simulink model "IntegratedSteamNetworkSimulation"  (R2022b)
settings: Solver=ode4  StartTime=0  StopTime=1000  FixedStep=0.5  MaxStep=1  MinStep=1e-3  EnableMultiTasking=on
values from neighbouring files (symbols this model uses):
  Attemp1_PB = 334.14047    [BoilerParam.m]
  Attemp1_RB = 332.70172955    [BoilerParam.m]
  Attemp2_PB = 426.4464    [BoilerParam.m]
  Attemp2_RB = 423.6721137    [BoilerParam.m]
  Attempflow_init = 0    [BoilerParam.m]
  Attempflow_SS = 11355    [BoilerParam.m]
  Attempflow_SSRB = 2.3*11355    (= 26116.5)    [BoilerParam.m]
  FG_flow_RB = 2.3*FGFlow_SS    (= 420210)    [BoilerParam.m]
  FGFlow_SS = 182700    [BoilerParam.m]
  hf = u(3)    [Boiler3.m]    (also in Boiler4.m; BoilerParam.m = 900000)
  phin = 6.21000008802327    (= 6.21000008802)    [BoilerParam.m]
  qfsteadystate = 73.2301    [BoilerParam.m]
  qfsteadystate2 = 31.5677    [BoilerParam.m]
  Qsteadystate = 1.374070083420811e+008    (= 137407008.342)    [BoilerParam.m]
  Qsteadystate2 = 5.9194e+007    (= 59194000)    [BoilerParam.m]
  TFG_out1_initPB = 432.2968    [BoilerParam.m]
  TFG_out1_initRB = 434.8845734    [BoilerParam.m]
  TFG_out2_initPB = 483.8618    [BoilerParam.m]
  TFG_out2_initRB = 486.31627357    [BoilerParam.m]
  TFG_out3_initPB = 543.7293    [BoilerParam.m]
  TFG_out3_initRB = 545.8638828    [BoilerParam.m]
  TFG_out4_initPB = 611.0105    [BoilerParam.m]
  TFG_out4_initRB = 612.6928895    [BoilerParam.m]
  TFG_out5_initPB = 684.8106    [BoilerParam.m]
  TFG_out5_initRB = 685.9654778    [BoilerParam.m]
  TFG_out6_initPB = 764.5389    [BoilerParam.m]
  TFG_out6_initRB = 765.12376925    [BoilerParam.m]
  Ts_out1_init_PB = 303.33953    [BoilerParam.m]
  Ts_out1_init_RB = 302.2065815    [BoilerParam.m]
  Ts_out2_init_PB = 334.14047    [BoilerParam.m]
  Ts_out2_init_RB = 332.70172955    [BoilerParam.m]
  Ts_out3_init_PB = 375.4672    [BoilerParam.m]
  Ts_out3_init_RB = 373.4655693    [BoilerParam.m]
  Ts_out4_init_PB = 426.4464    [BoilerParam.m]
  Ts_out4_init_RB = 423.6721137    [BoilerParam.m]
  Ts_out5_init_PB = 485.4202    [BoilerParam.m]
  Ts_out5_init_RB = 481.745302    [BoilerParam.m]
  Ts_out6_init_PB = 550.8115    [BoilerParam.m]
  Ts_out6_init_RB = 546.1691598    [BoilerParam.m]
  X0 = [106.953303000225 ... (first row only)    [BoilerParam.m]
  X02 = [39.2837325596915 ... (first row only)    [BoilerParam.m]
undefined symbols (not defined in the file or in its folder): Param, Param2, Param3, Param4, Param5, Param6
libraries: slpidlib x1
(part 1 of 2)
settings Model: Creator=aitai  LastModifiedBy=acer
settings DataIOCC: LimitDataPoints=on  SaveFinalState=on  SaveFormat=StructureWithTime  SignalLoggingSaveFormat=ModelDataLogs  ReturnWorkspaceOutputs=off  Refine=5
settings OptimizationCC: BlockReduction=off  BooleanDataType=off  BufferReuse=off  InitFltsAndDblsToZero=on  LifeSpan=inf
settings DebuggingCC: AlgebraicLoopMsg=none  SaveWithParameterizedLinksMsg=none  UnderspecifiedInitializationDetection=Classic  MergeDetectMultiDrivingBlocksExec=none  SignalResolutionControl=TryResolveAllWithWarning  MultiTaskDSMMsg=warning  MultiTaskCondExecSysMsg=none  SFUnexpectedBacktrackingDiag=warning  SFNoUnconditionalDefaultTransitionDiag=warning  SFExecutionAtInitializationDiag=none  SFMachineParentedDataDiag=warning  ArithmeticOperatorsInVariantConditions=warning
settings HardwareCC: ProdBitPerPointer=32  ProdBitPerSizeT=32  ProdBitPerPtrDiffT=32  ProdLargestAtomicFloat=None  ProdIntDivRoundTo=Undefined  ProdEndianess=Unspecified  ProdWordSize=32  ProdHWDeviceType=32-bit Generic  TargetUnknown=on
settings ModelReferenceCC: EnableRefExpFcnMdlSchedulingChecks=on  PropagateSignalLabelsOutOfModel=off
settings RTWCC: DLArmComputeVersion=19.05
settings CodeAppCC: StateflowObjectComments=on
settings GRTTargetCC: TargetFcnLib=ansi_tfl_tmw.mat  TargetLangStandard=C89/C90 (ANSI)  ModelReferenceCompliant=off  CombineOutputUpdateFcns=off  MatFileLogging=off  GRTInterface=on
settings ConfigComp: CovMetricSettings=dw  CovSaveCumulativeToWorkspaceVar=on  CovSaveSingleToWorkspaceVar=on

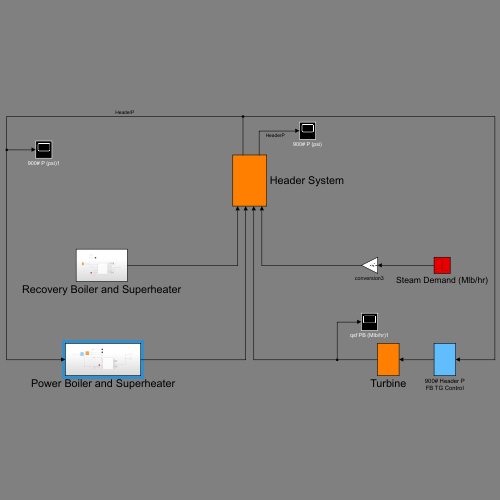
[thumbnail: Simulink's stored preview of the top-level diagram]
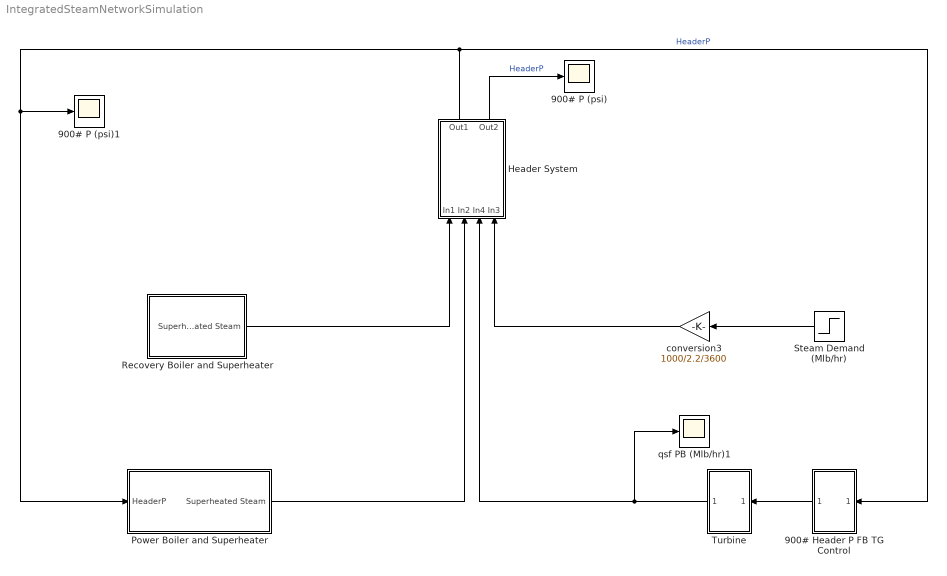
== system IntegratedSteamNetworkSimulation ==
  900# Header P FB TG Control : Subsystem
      mask Display: disp('')
  900# P (psi) : Scope
  900# P (psi)1 : Scope
  Header System : Subsystem
      mask Display: disp('')
  Power Boiler and Superheater : Subsystem
  Recovery Boiler and Superheater : Subsystem
  Steam Demand (Mlb/hr) : Step  Time=50  Before=240  After=210  SampleTime=0  VectorParams1D=off
  Turbine : Subsystem
      mask Display: disp('')
  conversion3 : Gain  Gain=1000/2.2/3600  SaturateOnIntegerOverflow=on  OutDataTypeStr=Inherit: Same as input  ParamDataTypeStr=Inherit: Same as input
  qsf PB (Mlb/hr)1 : Scope
  wires:
  Header System/1(Out1) -> 900# P (psi)1/1, Power Boiler and Superheater/1(HeaderP), 900# Header P FB TG Control/1(In1)  "HeaderP"
  Turbine/1(Out1) -> Header System/3(In4), qsf PB (Mlb/hr)1/1
  Steam Demand (Mlb/hr)/1 -> conversion3/1
  Header System/2(Out2) -> 900# P (psi)/1  "HeaderP"
  conversion3/1 -> Header System/4(In3)
  900# Header P FB TG Control/1(Out1) -> Turbine/1(In1)
  Power Boiler and Superheater/1(Superheated Steam) -> Header System/2(In2)
  Recovery Boiler and Superheater/1(Superheated Steam) -> Header System/1(In1)

== system IntegratedSteamNetworkSimulation/900# Header P FB TG Control ==
  In1 : Inport
  1/Ti1 : Gain  Gain=0.01  SaturateOnIntegerOverflow=on  OutDataTypeStr=Inherit: Same as input  ParamDataTypeStr=Inherit: Same as input
  900#  P Setpoint (psi) : Constant  Value=900
  Integrator1 : Integrator
  Kc1 : Gain  Gain=45  SaturateOnIntegerOverflow=on  OutDataTypeStr=Inherit: Same as input  ParamDataTypeStr=Inherit: Same as input
  P action1 : Gain  SaturateOnIntegerOverflow=on  OutDataTypeStr=Inherit: Same as input  ParamDataTypeStr=Inherit: Same as input
  Real Output from CO : Gain  Gain=0.01  SaturateOnIntegerOverflow=on  OutDataTypeStr=Inherit: Same as input  ParamDataTypeStr=Inherit: Same as input
  Sum2 : Sum  Inputs=|++  InputSameDT=on  SaturateOnIntegerOverflow=on  OutDataTypeStr=Inherit: Same as first input
  Sum3 : Sum  Inputs=|+-  InputSameDT=on  SaturateOnIntegerOverflow=on  OutDataTypeStr=Inherit: Same as first input
  Unit Delay : UnitDelay  SampleTime=-1  HasFrameUpgradeWarning=on
  conversion : Gain  Gain=6.21e6/900  SaturateOnIntegerOverflow=on  OutDataTypeStr=Inherit: Same as input  ParamDataTypeStr=Inherit: Same as input
  error as % of SP : Gain  Gain=100/6.21e6  SaturateOnIntegerOverflow=on  OutDataTypeStr=Inherit: Same as input  ParamDataTypeStr=Inherit: Same as input
  Out1 : Outport
  wires:
  1/Ti1/1 -> Integrator1/1
  Sum2/1 -> Kc1/1
  P action1/1 -> Sum2/1
  Integrator1/1 -> Sum2/2
  error as % of SP/1 -> 1/Ti1/1, P action1/1
  Kc1/1 -> Real Output from CO/1
  In1/1 -> Sum3/2
  900#  P Setpoint (psi)/1 -> conversion/1
  Sum3/1 -> error as % of SP/1
  Real Output from CO/1 -> Unit Delay/1
  conversion/1 -> Sum3/1
  Unit Delay/1 -> Out1/1

== system IntegratedSteamNetworkSimulation/Header System ==
  In1 : Inport
  In2 : Inport  Port=2
  In4 : Inport  Port=3
  In3 : Inport  Port=4
  " " : Gain  Gain=1e6  SaturateOnIntegerOverflow=on  OutDataTypeStr=Inherit: Same as input  ParamDataTypeStr=Inherit: Same as input
  Hdr : S-Function  FunctionName=hdr  Parameters=Param,phin  SFunctionDeploymentMode=off  EnableBusSupport=off
  Mux : Mux
  conversion : Gain  Gain=1/6.9e3  SaturateOnIntegerOverflow=on  OutDataTypeStr=Inherit: Same as input  ParamDataTypeStr=Inherit: Same as input
  Out1 : Outport
  Out2 : Outport  Port=2
  wires:
  In1/1 -> Mux/1
  In2/1 -> Mux/2
  In3/1 -> Mux/3
  In4/1 -> Mux/4
  Hdr/1 -> " "/1
  Mux/1 -> Hdr/1  "kg/s"
  " "/1 -> Out1/1, conversion/1  "Pa"
  conversion/1 -> Out2/1  "Psil"

== system IntegratedSteamNetworkSimulation/Power Boiler and Superheater ==
  note: s
  HeaderP : Inport
  900# Header P FB PB Control : Subsystem
      mask Display: disp('')
  FG Flow : Step  Before=FGFlow_SS  After=FGFlow_SS  SampleTime=0
  FG Temp : Scope  NumInputPorts=6
  Gain : Gain  Gain=FGFlow_SS
  PB Superheater : Subsystem
  Power Boiler : Subsystem
      mask Display: disp('')
  SH Steam Flow : Scope
  SH Steam Temp : Scope  NumInputPorts=8
  Scope6 : Scope
  Sum : Sum  Inputs=|++
  U1 : Step  Time=50000  Before=1.6  After=1.5  SampleTime=0
  conversion2 : Gain  Gain=2.2*3600/1000  SaturateOnIntegerOverflow=on  OutDataTypeStr=Inherit: Same as input  ParamDataTypeStr=Inherit: Same as input
  conversion4 : Gain  Gain=3600  SaturateOnIntegerOverflow=on  OutDataTypeStr=Inherit: Same as input  ParamDataTypeStr=Inherit: Same as input
  qsf PB (Mlb/hr) : Scope
  qsf PB (kg/s) : Scope
  Superheated Steam : Outport
  wires:
  conversion4/1 -> PB Superheater/2(Steamflowboiler)  "kg/hr"
  U1/1 -> PB Superheater/3(U-Value)
  PB Superheater/8(Ts_Out6) -> SH Steam Temp/8
  PB Superheater/9(SteamflowOut SH) -> Superheated Steam/1, SH Steam Flow/1  "Superheated Steam"
  HeaderP/1 -> 900# Header P FB PB Control/1(In1)
  PB Superheater/7(Ts_Out5) -> SH Steam Temp/7
  Power Boiler/1(qsf) -> conversion4/1, qsf PB (kg/s)/1, conversion2/1  "Saturated Steam"
  PB Superheater/6(Ts_OutAttemp2) -> SH Steam Temp/6
  PB Superheater/4(Ts_Out3) -> SH Steam Temp/4
  PB Superheater/13(TFG_Out4) -> FG Temp/4
  PB Superheater/1(Ts_out1) -> SH Steam Temp/1
  PB Superheater/11(TFG_Out2) -> FG Temp/2
  Power Boiler/2(PB_p) -> PB Superheater/1(Boiler Pressure)  "PB_P (Psi)"
  PB Superheater/2(Ts_Out2) -> SH Steam Temp/2
  900# Header P FB PB Control/1(Out1) -> Power Boiler/1(Delta Q)
  conversion2/1 -> qsf PB (Mlb/hr)/1
  PB Superheater/14(TFG_Out5) -> FG Temp/5
  PB Superheater/5(Ts_Out4) -> SH Steam Temp/5
  PB Superheater/10(TFG_Out1) -> FG Temp/1
  FG Flow/1 -> Sum/2
  PB Superheater/3(Ts_OutAttemp1) -> SH Steam Temp/3
  PB Superheater/12(TFG_Out3) -> FG Temp/3
  PB Superheater/15(TFG_Out6) -> FG Temp/6
  900# Header P FB PB Control/2(Output) -> Gain/1
  Sum/1 -> Scope6/1, PB Superheater/4(FG_flow)
  Gain/1 -> Sum/1

== system IntegratedSteamNetworkSimulation/Recovery Boiler and Superheater ==
  FG Flow1 : Step  Before=FG_flow_RB  After=FG_flow_RB  SampleTime=0
  FG Temp : Scope  NumInputPorts=6
  RB Superheater : Subsystem
  Recovery Boiler : Subsystem
      mask Display: disp('')
  SH Steam Temp : Scope  NumInputPorts=8
  Scope2 : Scope
  Scope4 : Scope
  U2 : Step  Time=50000  Before=1.6  After=1.5  SampleTime=0
  conversion1 : Gain  Gain=2.2*3600/1000  SaturateOnIntegerOverflow=on  OutDataTypeStr=Inherit: Same as input  ParamDataTypeStr=Inherit: Same as input
  conversion5 : Gain  Gain=3600  SaturateOnIntegerOverflow=on  OutDataTypeStr=Inherit: Same as input  ParamDataTypeStr=Inherit: Same as input
  qsf RB (Mlb/hr) : Scope
  Superheated Steam : Outport
  wires:
  RB Superheater/14(TFG_Out5) -> FG Temp/5
  Recovery Boiler/1(qsf) -> conversion5/1, Scope2/1, conversion1/1  "Saturated Steam"
  conversion1/1 -> qsf RB (Mlb/hr)/1
  RB Superheater/4(Ts_Out3) -> SH Steam Temp/4
  RB Superheater/15(TFG_Out6) -> FG Temp/6
  RB Superheater/5(Ts_Out4) -> SH Steam Temp/5
  RB Superheater/6(Ts_OutAttemp2) -> SH Steam Temp/6
  RB Superheater/2(Ts_Out2) -> SH Steam Temp/2
  RB Superheater/3(Ts_OutAttemp1) -> SH Steam Temp/3
  RB Superheater/11(TFG_Out2) -> FG Temp/2
  RB Superheater/8(Ts_Out6) -> SH Steam Temp/8
  RB Superheater/7(Ts_Out5) -> SH Steam Temp/7
  RB Superheater/9(SteamflowOut SH) -> Superheated Steam/1, Scope4/1
  conversion5/1 -> RB Superheater/2(Steamflowboiler)  "kg/hr"
  RB Superheater/1(Ts_out1) -> SH Steam Temp/1
  FG Flow1/1 -> RB Superheater/4(FG_flow)
  RB Superheater/13(TFG_Out4) -> FG Temp/4
  RB Superheater/10(TFG_Out1) -> FG Temp/1
  RB Superheater/12(TFG_Out3) -> FG Temp/3
  Recovery Boiler/2(RB_P) -> RB Superheater/1(Boiler Pressure)  "RB_P"
  U2/1 -> RB Superheater/3(U-Value)

== system IntegratedSteamNetworkSimulation/Turbine ==
  In1 : Inport
  Sum4 : Sum  Inputs=|-+  InputSameDT=on  SaturateOnIntegerOverflow=on  OutDataTypeStr=Inherit: Same as first input
  TG Dynamics : TransferFcn  Denominator=[5 1]
  TG SS Demand (Mlb/hr) : Constant  Value=590
  conversion : Gain  Gain=1000/2.2/3600  SaturateOnIntegerOverflow=on  OutDataTypeStr=Inherit: Same as input  ParamDataTypeStr=Inherit: Same as input
  Out1 : Outport
  wires:
  TG SS Demand (Mlb/hr)/1 -> conversion/1
  TG Dynamics/1 -> Sum4/1
  Sum4/1 -> Out1/1
  In1/1 -> TG Dynamics/1
  conversion/1 -> Sum4/2

== system IntegratedSteamNetworkSimulation/Power Boiler and Superheater/900# Header P FB PB Control ==
  In1 : Inport
  1/Ti1 : Gain  Gain=0.001  SaturateOnIntegerOverflow=on  OutDataTypeStr=Inherit: Same as input  ParamDataTypeStr=Inherit: Same as input
  900#  P Setpoint (psi) : Constant  Value=900
  Constant : Constant  Value=Qsteadystate2
  Divide : Product  Inputs=*/
  Integrator1 : Integrator
  Kc1 : Gain  Gain=15  SaturateOnIntegerOverflow=on  OutDataTypeStr=Inherit: Same as input  ParamDataTypeStr=Inherit: Same as input
  P action1 : Gain  SaturateOnIntegerOverflow=on  OutDataTypeStr=Inherit: Same as input  ParamDataTypeStr=Inherit: Same as input
  Real Output from CO : Gain  Gain=Qsteadystate2/100  SaturateOnIntegerOverflow=on  OutDataTypeStr=Inherit: Same as input  ParamDataTypeStr=Inherit: Same as input
  Scope : Scope  NumInputPorts=2
  Scope1 : Scope
  Sum2 : Sum  Inputs=|++  InputSameDT=on  SaturateOnIntegerOverflow=on  OutDataTypeStr=Inherit: Same as first input
  Sum3 : Sum  Inputs=|+-  InputSameDT=on  SaturateOnIntegerOverflow=on  OutDataTypeStr=Inherit: Same as first input
  conversion : Gain  Gain=6.21e6/900  SaturateOnIntegerOverflow=on  OutDataTypeStr=Inherit: Same as input  ParamDataTypeStr=Inherit: Same as input
  error as % of SP : Gain  Gain=100/6.21e6  SaturateOnIntegerOverflow=on  OutDataTypeStr=Inherit: Same as input  ParamDataTypeStr=Inherit: Same as input
  Out1 : Outport
  Output : Outport  Port=2
  wires:
  1/Ti1/1 -> Integrator1/1
  Sum2/1 -> Kc1/1
  P action1/1 -> Sum2/1
  Integrator1/1 -> Sum2/2
  error as % of SP/1 -> 1/Ti1/1, P action1/1
  Kc1/1 -> Scope/1, Real Output from CO/1
  In1/1 -> Sum3/2
  900#  P Setpoint (psi)/1 -> conversion/1
  Sum3/1 -> error as % of SP/1
  Real Output from CO/1 -> Divide/1, Out1/1, Scope/2
  conversion/1 -> Sum3/1
  Constant/1 -> Divide/2
  Divide/1 -> Scope1/1, Output/1

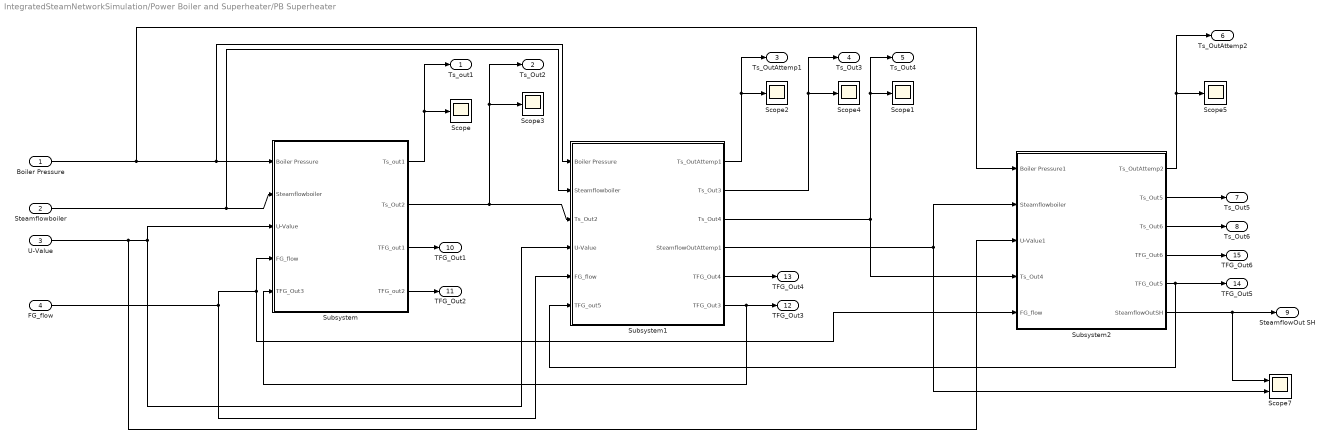
== system IntegratedSteamNetworkSimulation/Power Boiler and Superheater/PB Superheater ==
  Boiler Pressure : Inport
  Steamflowboiler : Inport  Port=2
  U-Value : Inport  Port=3
  FG_flow : Inport  Port=4
  Scope{,1..5} (6 alike) : Scope
  Scope7 : Scope  NumInputPorts=2
  Subsystem : Subsystem
  Subsystem1 : Subsystem
  Subsystem2 : Subsystem
  Ts_out1 : Outport
  Ts_Out2 : Outport  Port=2
  Ts_OutAttemp1 : Outport  Port=3
  Ts_Out3 : Outport  Port=4
  Ts_Out4 : Outport  Port=5
  Ts_OutAttemp2 : Outport  Port=6
  Ts_Out5 : Outport  Port=7
  Ts_Out6 : Outport  Port=8
  SteamflowOut SH : Outport  Port=9
  TFG_Out1 : Outport  Port=10
  TFG_Out2 : Outport  Port=11
  TFG_Out3 : Outport  Port=12
  TFG_Out4 : Outport  Port=13
  TFG_Out5 : Outport  Port=14
  TFG_Out6 : Outport  Port=15
  wires:
  Subsystem/1(Ts_out1) -> Ts_out1/1, Scope/1
  Steamflowboiler/1 -> Subsystem1/2(Steamflowboiler), Subsystem/2(Steamflowboiler)
  Boiler Pressure/1 -> Subsystem2/1(Boiler Pressure1), Subsystem/1(Boiler Pressure), Subsystem1/1(Boiler Pressure)
  Subsystem/2(Ts_Out2) -> Subsystem1/3(Ts_Out2), Ts_Out2/1, Scope3/1
  Subsystem1/1(Ts_OutAttemp1) -> Ts_OutAttemp1/1, Scope2/1
  Subsystem1/2(Ts_Out3) -> Ts_Out3/1, Scope4/1
  Subsystem1/3(Ts_Out4) -> Scope1/1, Ts_Out4/1, Subsystem2/4(Ts_Out4)
  U-Value/1 -> Subsystem2/3(U-Value1), Subsystem1/4(U-Value), Subsystem/3(U-Value)
  Subsystem2/1(Ts_OutAttemp2) -> Scope5/1, Ts_OutAttemp2/1
  Subsystem2/2(Ts_Out5) -> Ts_Out5/1
  Subsystem2/3(Ts_Out6) -> Ts_Out6/1
  Subsystem2/6(SteamflowOutSH) -> Scope7/1, SteamflowOut SH/1
  Subsystem1/4(SteamflowOutAttemp1) -> Subsystem2/2(Steamflowboiler), Scope7/2
  FG_flow/1 -> Subsystem2/5(FG_flow), Subsystem/4(FG_flow), Subsystem1/5(FG_flow)
  Subsystem1/6(TFG_Out3) -> Subsystem/5(TFG_Out3), TFG_Out3/1
  Subsystem2/5(TFG_Out5) -> Subsystem1/6(TFG_out5), TFG_Out5/1
  Subsystem/3(TFG_out1) -> TFG_Out1/1
  Subsystem/4(TFG_out2) -> TFG_Out2/1
  Subsystem1/5(TFG_Out4) -> TFG_Out4/1
  Subsystem2/4(TFG_Out6) -> TFG_Out6/1

== system IntegratedSteamNetworkSimulation/Power Boiler and Superheater/Power Boiler ==
  Delta Q : Inport
  3 Element Level Control System : Subsystem
  PB feed water (Mlb/hr) : Scope
  PB level (in) : Scope
  PB pressure (psi) : Scope
  Power Boiler : Subsystem
  qsf : Outport
  PB_p : Outport  Port=2
  wires:
  Power Boiler/2(qsf) -> qsf/1, 3 Element Level Control System/2(In2)
  Power Boiler/1(l) -> PB level (in)/1, 3 Element Level Control System/1(In1)
  Delta Q/1 -> Power Boiler/2(Delta Q)
  Power Boiler/3(PB p) -> PB_p/1, PB pressure (psi)/1
  Power Boiler/4(qf) -> PB feed water (Mlb/hr)/1
  3 Element Level Control System/1(Delta qf) -> Power Boiler/1(Delta qf)

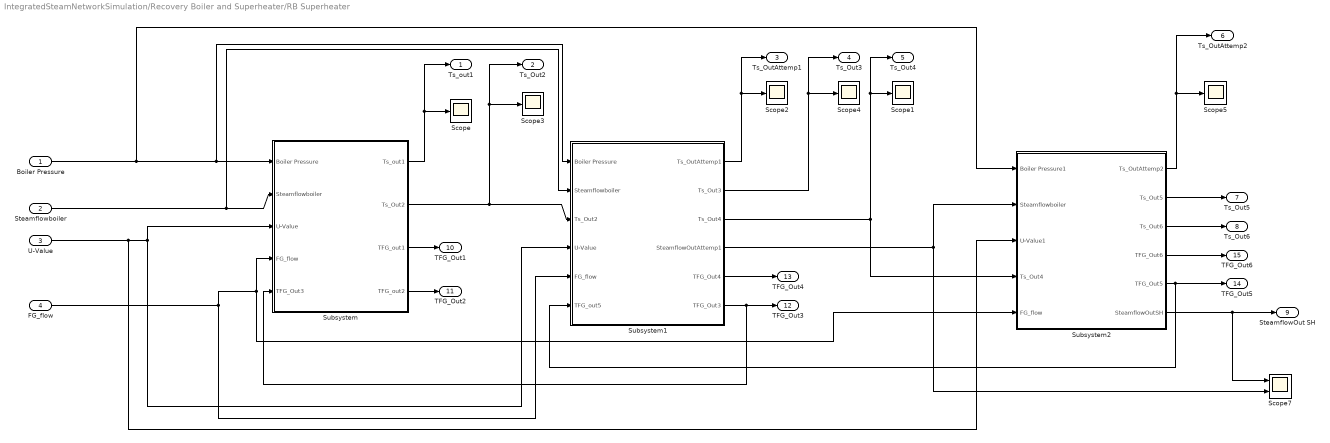
== system IntegratedSteamNetworkSimulation/Recovery Boiler and Superheater/RB Superheater ==
  Boiler Pressure : Inport
  Steamflowboiler : Inport  Port=2
  U-Value : Inport  Port=3
  FG_flow : Inport  Port=4
  Scope{,1..5} (6 alike) : Scope
  Scope7 : Scope  NumInputPorts=2
  Subsystem : Subsystem
  Subsystem1 : Subsystem
  Subsystem2 : Subsystem
  Ts_out1 : Outport
  Ts_Out2 : Outport  Port=2
  Ts_OutAttemp1 : Outport  Port=3
  Ts_Out3 : Outport  Port=4
  Ts_Out4 : Outport  Port=5
  Ts_OutAttemp2 : Outport  Port=6
  Ts_Out5 : Outport  Port=7
  Ts_Out6 : Outport  Port=8
  SteamflowOut SH : Outport  Port=9
  TFG_Out1 : Outport  Port=10
  TFG_Out2 : Outport  Port=11
  TFG_Out3 : Outport  Port=12
  TFG_Out4 : Outport  Port=13
  TFG_Out5 : Outport  Port=14
  TFG_Out6 : Outport  Port=15
  wires:
  Subsystem/1(Ts_out1) -> Ts_out1/1, Scope/1
  Steamflowboiler/1 -> Subsystem1/2(Steamflowboiler), Subsystem/2(Steamflowboiler)
  Boiler Pressure/1 -> Subsystem2/1(Boiler Pressure1), Subsystem/1(Boiler Pressure), Subsystem1/1(Boiler Pressure)
  Subsystem/2(Ts_Out2) -> Subsystem1/3(Ts_Out2), Ts_Out2/1, Scope3/1
  Subsystem1/1(Ts_OutAttemp1) -> Ts_OutAttemp1/1, Scope2/1
  Subsystem1/2(Ts_Out3) -> Ts_Out3/1, Scope4/1
  Subsystem1/3(Ts_Out4) -> Scope1/1, Ts_Out4/1, Subsystem2/4(Ts_Out4)
  U-Value/1 -> Subsystem2/3(U-Value1), Subsystem1/4(U-Value), Subsystem/3(U-Value)
  Subsystem2/1(Ts_OutAttemp2) -> Scope5/1, Ts_OutAttemp2/1
  Subsystem2/2(Ts_Out5) -> Ts_Out5/1
  Subsystem2/3(Ts_Out6) -> Ts_Out6/1
  Subsystem2/6(SteamflowOutSH) -> Scope7/1, SteamflowOut SH/1
  Subsystem1/4(SteamflowOutAttemp1) -> Subsystem2/2(Steamflowboiler), Scope7/2
  FG_flow/1 -> Subsystem2/5(FG_flow), Subsystem/4(FG_flow), Subsystem1/5(FG_flow)
  Subsystem1/6(TFG_Out3) -> Subsystem/5(TFG_Out3), TFG_Out3/1
  Subsystem2/5(TFG_Out5) -> Subsystem1/6(TFG_out5), TFG_Out5/1
  Subsystem/3(TFG_out1) -> TFG_Out1/1
  Subsystem/4(TFG_out2) -> TFG_Out2/1
  Subsystem1/5(TFG_Out4) -> TFG_Out4/1
  Subsystem2/4(TFG_Out6) -> TFG_Out6/1

== system IntegratedSteamNetworkSimulation/Recovery Boiler and Superheater/Recovery Boiler ==
  3 Element Level Control System : Subsystem
  Firing Rate Change (% of nominal) : Step  Before=Qsteadystate*0  After=Qsteadystate*0  SampleTime=0
  RB Pressure (Psi) : Scope
  RB feed water (Mlb/hr) : Scope
  RB level (in) : Scope
  Recovery Boiler : Subsystem
  Scope : Scope
  qsf : Outport
  RB_P : Outport  Port=2
  wires:
  Recovery Boiler/2(qsf) -> qsf/1, 3 Element Level Control System/2(In2)
  Recovery Boiler/1(l) -> RB level (in)/1, 3 Element Level Control System/1(In1)
  Firing Rate Change (% of nominal)/1 -> Recovery Boiler/2(Delta Q)
  Recovery Boiler/3(RB p) -> RB Pressure (Psi)/1, RB_P/1
  Recovery Boiler/4(qf) -> RB feed water (Mlb/hr)/1
  3 Element Level Control System/1(Delta qf) -> Recovery Boiler/1(Delta qf), Scope/1

== system IntegratedSteamNetworkSimulation/Power Boiler and Superheater/PB Superheater/Subsystem ==
  Boiler Pressure : Inport
  Steamflowboiler : Inport  Port=2
  U-Value : Inport  Port=3
  FG_flow : Inport  Port=4
  TFG_Out3 : Inport  Port=5
  Demux : Demux  Outputs=1
  Demux1 : Demux  Outputs=2
  Demux2 : Demux  Outputs=2
  Mux : Mux
  Mux1 : Mux  Inputs=5
  Mux2 : Mux
  Mux3 : Mux
  Scope{1..4} (4 alike) : Scope
  Superheater1_FG : S-Function  FunctionName=PBsuperheater1_FGDyn  Parameters=Param5,TFG_out1_initPB  SFunctionDeploymentMode=off  EnableBusSupport=off
  Superheater1_Steam : S-Function  FunctionName=PBsuperheater1  Parameters=Param3,Ts_out1_init_PB  SFunctionDeploymentMode=off  EnableBusSupport=off
  Superheater2_FG : S-Function  FunctionName=PBsuperheater2_FGDyn  Parameters=Param5,TFG_out2_initPB  SFunctionDeploymentMode=off  EnableBusSupport=off
  Superheater2_Steam : S-Function  FunctionName=PBsuperheater2  Parameters=Param3,Ts_out2_init_PB  SFunctionDeploymentMode=off  EnableBusSupport=off
  Ts_out1 : Outport
  Ts_Out2 : Outport  Port=2
  TFG_out1 : Outport  Port=3
  TFG_out2 : Outport  Port=4
  wires:
  Boiler Pressure/1 -> Mux/1, Mux1/1
  Superheater1_Steam/1 -> Demux/1
  Mux/1 -> Superheater1_Steam/1
  Steamflowboiler/1 -> Mux/2, Mux1/2
  Mux1/1 -> Superheater2_Steam/1
  Demux/1 -> Mux3/4, Mux1/4, Ts_out1/1
  U-Value/1 -> Mux1/3, Mux2/3, Mux3/3, Mux/3
  Superheater1_FG/1 -> Demux2/1
  Demux2/2 -> Scope2/1  "Q (kW)"
  Demux1/2 -> Scope4/1  "Q (kW)"
  Demux2/1 -> Scope1/1, TFG_out1/1, Mux/4  "TFG_out1"
  TFG_Out3/1 -> Mux2/2
  Superheater2_Steam/1 -> Ts_Out2/1, Mux2/4
  FG_flow/1 -> Mux2/1, Mux3/1
  Demux1/1 -> Scope3/1, TFG_out2/1, Mux1/5, Mux3/2  "TFG_out2"
  Superheater2_FG/1 -> Demux1/1
  Mux3/1 -> Superheater1_FG/1
  Mux2/1 -> Superheater2_FG/1

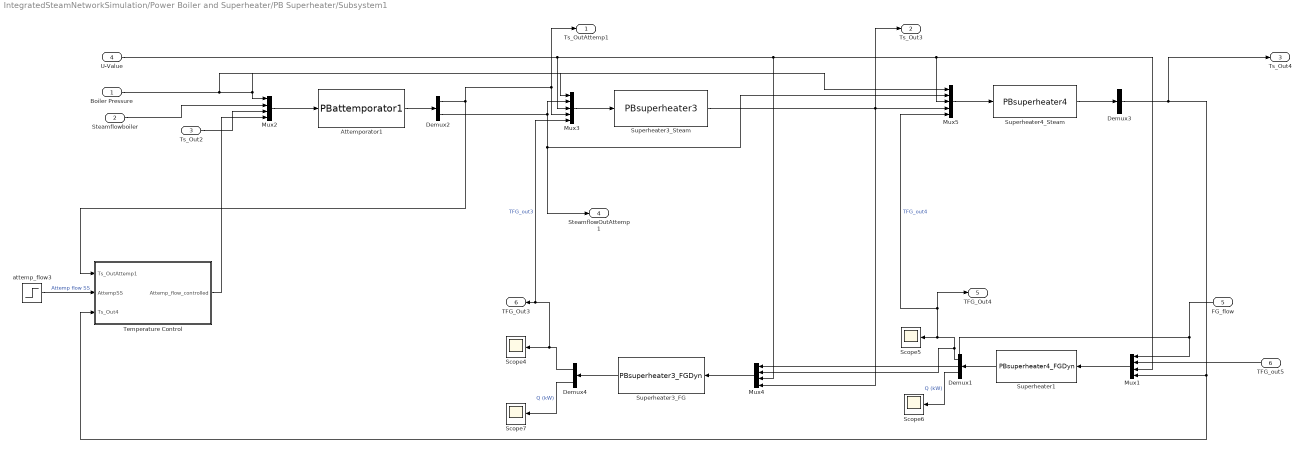
== system IntegratedSteamNetworkSimulation/Power Boiler and Superheater/PB Superheater/Subsystem1 ==
  Boiler Pressure : Inport
  Steamflowboiler : Inport  Port=2
  Ts_Out2 : Inport  Port=3
  U-Value : Inport  Port=4
  FG_flow : Inport  Port=5
  TFG_out5 : Inport  Port=6
  Attemporator1 : S-Function  FunctionName=PBattemporator1  Parameters=Param3, Attemp1_PB  SFunctionDeploymentMode=off  EnableBusSupport=off
  Demux1 : Demux  Outputs=2
  Demux2 : Demux  Outputs=2
  Demux3 : Demux  Outputs=1
  Demux4 : Demux  Outputs=2
  Mux1 : Mux
  Mux2 : Mux
  Mux3 : Mux  Inputs=5
  Mux4 : Mux
  Mux5 : Mux  Inputs=5
  Scope{4..7} (4 alike) : Scope
  Superheater1 : S-Function  FunctionName=PBsuperheater4_FGDyn  Parameters=Param5,TFG_out4_initPB  SFunctionDeploymentMode=off  EnableBusSupport=off
  Superheater3_FG : S-Function  FunctionName=PBsuperheater3_FGDyn  Parameters=Param5,TFG_out3_initPB  SFunctionDeploymentMode=off  EnableBusSupport=off
  Superheater3_Steam : S-Function  FunctionName=PBsuperheater3  Parameters=Param3,Ts_out3_init_PB  SFunctionDeploymentMode=off  EnableBusSupport=off
  Superheater4_Steam : S-Function  FunctionName=PBsuperheater4  Parameters=Param3,Ts_out4_init_PB  SFunctionDeploymentMode=off  EnableBusSupport=off
  Temperature Control : Subsystem
  attemp_flow3 : Step  Time=100  Before=Attempflow_init  After=Attempflow_init  SampleTime=0
  Ts_OutAttemp1 : Outport
  Ts_Out3 : Outport  Port=2
  Ts_Out4 : Outport  Port=3
  SteamflowOutAttemp1 : Outport  Port=4
  TFG_Out4 : Outport  Port=5
  TFG_Out3 : Outport  Port=6
  wires:
  Mux2/1 -> Attemporator1/1
  Superheater4_Steam/1 -> Demux3/1
  Mux3/1 -> Superheater3_Steam/1
  Mux5/1 -> Superheater4_Steam/1
  Attemporator1/1 -> Demux2/1
  Demux2/2 -> Mux3/2, SteamflowOutAttemp1/1, Mux5/2
  Boiler Pressure/1 -> Mux5/1, Mux3/1, Mux2/1
  Steamflowboiler/1 -> Mux2/2
  Ts_Out2/1 -> Mux2/3
  attemp_flow3/1 -> Temperature Control/2(AttempSS)  "Attemp flow SS"
  Demux2/1 -> Ts_OutAttemp1/1, Mux3/4, Temperature Control/1(Ts_OutAttemp1)
  Temperature Control/1(Attemp_flow_controlled) -> Mux2/4
  Demux4/1 -> Mux3/5, TFG_Out3/1, Scope4/1  "TFG_out3"
  TFG_out5/1 -> Mux1/2
  Superheater3_FG/1 -> Demux4/1
  Demux1/1 -> Mux4/2, Mux5/5, TFG_Out4/1, Scope5/1  "TFG_out4"
  Superheater1/1 -> Demux1/1
  Demux3/1 -> Temperature Control/3(Ts_Out4), Mux1/4, Ts_Out4/1
  Demux1/2 -> Scope6/1  "Q (kW)"
  Superheater3_Steam/1 -> Mux4/4, Mux5/4, Ts_Out3/1
  U-Value/1 -> Mux3/3, Mux4/3, Mux5/3, Mux1/3
  Demux4/2 -> Scope7/1  "Q (kW)"
  FG_flow/1 -> Mux4/1, Mux1/1
  Mux4/1 -> Superheater3_FG/1
  Mux1/1 -> Superheater1/1

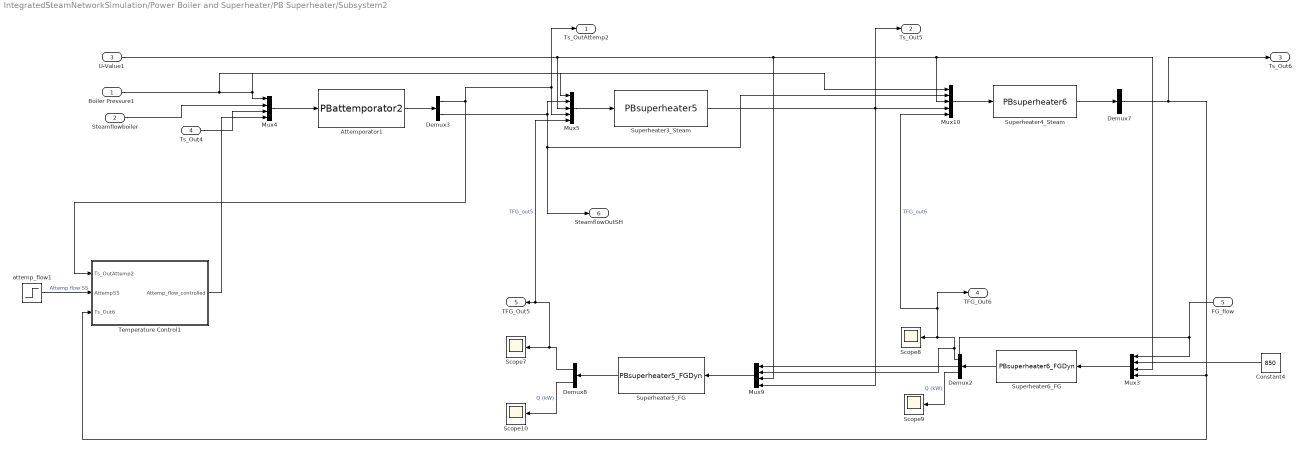
== system IntegratedSteamNetworkSimulation/Power Boiler and Superheater/PB Superheater/Subsystem2 ==
  Boiler Pressure1 : Inport
  Steamflowboiler : Inport  Port=2
  U-Value1 : Inport  Port=3
  Ts_Out4 : Inport  Port=4
  FG_flow : Inport  Port=5
  Attemporator1 : S-Function  FunctionName=PBattemporator2  Parameters=Param3,Attemp2_PB  SFunctionDeploymentMode=off  EnableBusSupport=off
  Constant4 : Constant  Value=850
  Demux2 : Demux  Outputs=2
  Demux3 : Demux  Outputs=2
  Demux7 : Demux  Outputs=1
  Demux8 : Demux  Outputs=2
  Mux10 : Mux  Inputs=5
  Mux3 : Mux
  Mux4 : Mux
  Mux5 : Mux  Inputs=5
  Mux9 : Mux
  Scope{7..10} (4 alike) : Scope
  Superheater3_Steam : S-Function  FunctionName=PBsuperheater5  Parameters=Param3,Ts_out5_init_PB  SFunctionDeploymentMode=off  EnableBusSupport=off
  Superheater4_Steam : S-Function  FunctionName=PBsuperheater6  Parameters=Param3,Ts_out6_init_PB  SFunctionDeploymentMode=off  EnableBusSupport=off
  Superheater5_FG : S-Function  FunctionName=PBsuperheater5_FGDyn  Parameters=Param5,TFG_out5_initPB  SFunctionDeploymentMode=off  EnableBusSupport=off
  Superheater6_FG : S-Function  FunctionName=PBsuperheater6_FGDyn  Parameters=Param5,TFG_out6_initPB  SFunctionDeploymentMode=off  EnableBusSupport=off
  Temperature Control1 : Subsystem
  attemp_flow1 : Step  Time=100  Before=Attempflow_init  After=Attempflow_init  SampleTime=0
  Ts_OutAttemp2 : Outport
  Ts_Out5 : Outport  Port=2
  Ts_Out6 : Outport  Port=3
  TFG_Out6 : Outport  Port=4
  TFG_Out5 : Outport  Port=5
  SteamflowOutSH : Outport  Port=6
  wires:
  Demux8/1 -> Mux5/5, TFG_Out5/1, Scope7/1  "TFG_out5"
  Demux3/1 -> Temperature Control1/1(Ts_OutAttemp2), Ts_OutAttemp2/1, Mux5/4
  Superheater5_FG/1 -> Demux8/1
  Superheater6_FG/1 -> Demux2/1
  Mux4/1 -> Attemporator1/1
  Constant4/1 -> Mux3/2
  Temperature Control1/1(Attemp_flow_controlled) -> Mux4/4
  Demux7/1 -> Temperature Control1/3(Ts_Out6), Mux3/4, Ts_Out6/1
  Demux3/2 -> Mux5/2, SteamflowOutSH/1, Mux10/2
  Demux8/2 -> Scope10/1  "Q (kW)"
  Mux9/1 -> Superheater5_FG/1
  FG_flow/1 -> Mux9/1, Mux3/1
  Demux2/2 -> Scope9/1  "Q (kW)"
  U-Value1/1 -> Mux5/3, Mux9/3, Mux10/3, Mux3/3
  Mux3/1 -> Superheater6_FG/1
  Superheater3_Steam/1 -> Mux9/4, Mux10/4, Ts_Out5/1
  Demux2/1 -> Mux9/2, Mux10/5, TFG_Out6/1, Scope8/1  "TFG_out6"
  Superheater4_Steam/1 -> Demux7/1
  attemp_flow1/1 -> Temperature Control1/2(AttempSS)  "Attemp flow SS"
  Mux5/1 -> Superheater3_Steam/1
  Ts_Out4/1 -> Mux4/3
  Boiler Pressure1/1 -> Mux10/1, Mux5/1, Mux4/1
  Steamflowboiler/1 -> Mux4/2
  Mux10/1 -> Superheater4_Steam/1
  Attemporator1/1 -> Demux3/1

== system IntegratedSteamNetworkSimulation/Power Boiler and Superheater/Power Boiler/3 Element Level Control System ==
  In1 : Inport
  In2 : Inport  Port=2
  Add1 : Sum  Inputs=+-
  Bias : Constant  Value=50
  FB Level Control : Subsystem
  FF Gain : Gain  SaturateOnIntegerOverflow=on  OutDataTypeStr=Inherit: Same as input  ParamDataTypeStr=Inherit: Same as input
  Level Setpoint (in) : Constant  Value=0.5
  Nominal : Step  Time=10  Before=qfsteadystate2  After=qfsteadystate2  SampleTime=0
  Real Output from CO : Gain  Gain=6  SaturateOnIntegerOverflow=on  OutDataTypeStr=Inherit: Same as input  ParamDataTypeStr=Inherit: Same as input
  Sum3 : Sum  Inputs=|++-  InputSameDT=on  SaturateOnIntegerOverflow=on  OutDataTypeStr=Inherit: Same as first input
  conversion : Gain  Gain=1000/2.2/3600  SaturateOnIntegerOverflow=on  OutDataTypeStr=Inherit: Same as input  ParamDataTypeStr=Inherit: Same as input
  conversion1 : Gain  Gain=1/(1000/2.2/3600)  SaturateOnIntegerOverflow=on  OutDataTypeStr=Inherit: Same as input  ParamDataTypeStr=Inherit: Same as input
  scaling : Gain  Gain=1/6  SaturateOnIntegerOverflow=on  OutDataTypeStr=Inherit: Same as input  ParamDataTypeStr=Inherit: Same as input
  Delta qf : Outport
  wires:
  In2/1 -> conversion1/1
  Level Setpoint (in)/1 -> FB Level Control/1(In1)
  In1/1 -> FB Level Control/2(In2)
  FB Level Control/1(Out1) -> Sum3/1
  Bias/1 -> Sum3/3
  Sum3/1 -> Real Output from CO/1
  Real Output from CO/1 -> conversion/1
  conversion1/1 -> scaling/1
  Add1/1 -> Delta qf/1
  scaling/1 -> FF Gain/1
  conversion/1 -> Add1/1
  Nominal/1 -> Add1/2
  FF Gain/1 -> Sum3/2

== system IntegratedSteamNetworkSimulation/Power Boiler and Superheater/Power Boiler/Power Boiler ==
  Delta qf : Inport
  Delta Q : Inport  Port=2
  Bias : Bias  Bias=-0.64  SaturateOnIntegerOverflow=off
  FireSide Dyn. : TransferFcn  Denominator=[5 1]
  Power Boiler : Subsystem
  Transport Delay : TransportDelay  DelayTime=10
  conversion : Gain  Gain=100/2.54  SaturateOnIntegerOverflow=on  OutDataTypeStr=Inherit: Same as input  ParamDataTypeStr=Inherit: Same as input
  conversion1 : Gain  Gain=1/6.9e3  SaturateOnIntegerOverflow=on  OutDataTypeStr=Inherit: Same as input  ParamDataTypeStr=Inherit: Same as input
  conversion2 : Gain  Gain=2.2*3600/1000  SaturateOnIntegerOverflow=on  OutDataTypeStr=Inherit: Same as input  ParamDataTypeStr=Inherit: Same as input
  l : Outport
  qsf : Outport  Port=2
  PB p : Outport  Port=3
  qf : Outport  Port=4
  wires:
  Delta qf/1 -> Power Boiler/1(In2)
  Power Boiler/2(Out1) -> qsf/1
  Transport Delay/1 -> FireSide Dyn./1
  Delta Q/1 -> Transport Delay/1
  FireSide Dyn./1 -> Power Boiler/2(In3)
  conversion/1 -> l/1
  Power Boiler/1(Out2) -> Bias/1
  Bias/1 -> conversion/1
  conversion1/1 -> PB p/1
  Power Boiler/3(Out3) -> conversion1/1
  Power Boiler/4(Out4) -> conversion2/1
  conversion2/1 -> qf/1

== system IntegratedSteamNetworkSimulation/Recovery Boiler and Superheater/RB Superheater/Subsystem ==
  Boiler Pressure : Inport
  Steamflowboiler : Inport  Port=2
  U-Value : Inport  Port=3
  FG_flow : Inport  Port=4
  TFG_Out3 : Inport  Port=5
  Demux : Demux  Outputs=1
  Demux1 : Demux  Outputs=2
  Demux2 : Demux  Outputs=2
  Mux : Mux
  Mux1 : Mux  Inputs=5
  Mux2 : Mux
  Mux3 : Mux
  Scope{1..4} (4 alike) : Scope
  Superheater1_FG : S-Function  FunctionName=RBsuperheater1_FGDyn  Parameters=Param6,TFG_out1_initRB  SFunctionDeploymentMode=off  EnableBusSupport=off
  Superheater1_Steam : S-Function  FunctionName=RBsuperheater1  Parameters=Param4,Ts_out1_init_RB  SFunctionDeploymentMode=off  EnableBusSupport=off
  Superheater2_FG : S-Function  FunctionName=RBsuperheater2_FGDyn  Parameters=Param6,TFG_out2_initRB  SFunctionDeploymentMode=off  EnableBusSupport=off
  Superheater2_Steam : S-Function  FunctionName=RBsuperheater2  Parameters=Param4,Ts_out2_init_RB  SFunctionDeploymentMode=off  EnableBusSupport=off
  Ts_out1 : Outport
  Ts_Out2 : Outport  Port=2
  TFG_out1 : Outport  Port=3
  TFG_out2 : Outport  Port=4
  wires:
  Boiler Pressure/1 -> Mux/1, Mux1/1
  Superheater1_Steam/1 -> Demux/1
  Mux/1 -> Superheater1_Steam/1
  Steamflowboiler/1 -> Mux/2, Mux1/2
  Mux1/1 -> Superheater2_Steam/1
  Demux/1 -> Mux3/4, Mux1/4, Ts_out1/1
  U-Value/1 -> Mux1/3, Mux2/3, Mux3/3, Mux/3
  Superheater1_FG/1 -> Demux2/1
  Demux2/2 -> Scope2/1  "Q (kW)"
  Demux1/2 -> Scope4/1  "Q (kW)"
  Demux2/1 -> Scope1/1, TFG_out1/1, Mux/4  "TFG_out1"
  TFG_Out3/1 -> Mux2/2
  Superheater2_Steam/1 -> Ts_Out2/1, Mux2/4
  FG_flow/1 -> Mux2/1, Mux3/1
  Demux1/1 -> Scope3/1, TFG_out2/1, Mux1/5, Mux3/2  "TFG_out2"
  Superheater2_FG/1 -> Demux1/1
  Mux3/1 -> Superheater1_FG/1
  Mux2/1 -> Superheater2_FG/1

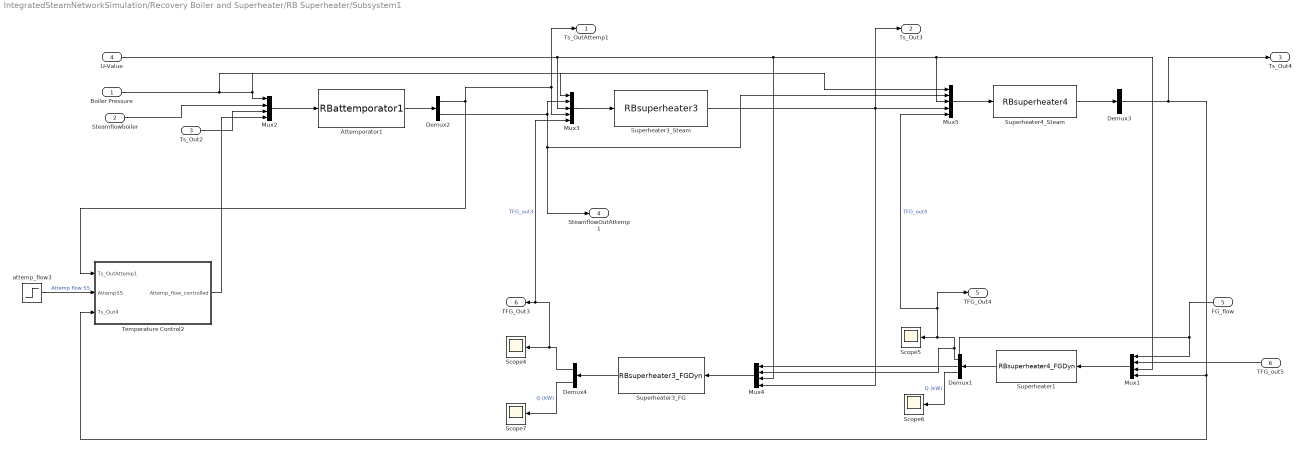
== system IntegratedSteamNetworkSimulation/Recovery Boiler and Superheater/RB Superheater/Subsystem1 ==
  Boiler Pressure : Inport
  Steamflowboiler : Inport  Port=2
  Ts_Out2 : Inport  Port=3
  U-Value : Inport  Port=4
  FG_flow : Inport  Port=5
  TFG_out5 : Inport  Port=6
  Attemporator1 : S-Function  FunctionName=RBattemporator1  Parameters=Param4, Attemp1_RB  SFunctionDeploymentMode=off  EnableBusSupport=off
  Demux1 : Demux  Outputs=2
  Demux2 : Demux  Outputs=2
  Demux3 : Demux  Outputs=1
  Demux4 : Demux  Outputs=2
  Mux1 : Mux
  Mux2 : Mux
  Mux3 : Mux  Inputs=5
  Mux4 : Mux
  Mux5 : Mux  Inputs=5
  Scope{4..7} (4 alike) : Scope
  Superheater1 : S-Function  FunctionName=RBsuperheater4_FGDyn  Parameters=Param6,TFG_out4_initRB  SFunctionDeploymentMode=off  EnableBusSupport=off
  Superheater3_FG : S-Function  FunctionName=RBsuperheater3_FGDyn  Parameters=Param6,TFG_out3_initRB  SFunctionDeploymentMode=off  EnableBusSupport=off
  Superheater3_Steam : S-Function  FunctionName=RBsuperheater3  Parameters=Param4,Ts_out3_init_RB  SFunctionDeploymentMode=off  EnableBusSupport=off
  Superheater4_Steam : S-Function  FunctionName=RBsuperheater4  Parameters=Param4,Ts_out4_init_RB  SFunctionDeploymentMode=off  EnableBusSupport=off
  Temperature Control2 : Subsystem
  attemp_flow3 : Step  Time=100  Before=Attempflow_init  After=Attempflow_init  SampleTime=0
  Ts_OutAttemp1 : Outport
  Ts_Out3 : Outport  Port=2
  Ts_Out4 : Outport  Port=3
  SteamflowOutAttemp1 : Outport  Port=4
  TFG_Out4 : Outport  Port=5
  TFG_Out3 : Outport  Port=6
  wires:
  Mux2/1 -> Attemporator1/1
  Superheater4_Steam/1 -> Demux3/1
  Mux3/1 -> Superheater3_Steam/1
  Mux5/1 -> Superheater4_Steam/1
  Attemporator1/1 -> Demux2/1
  Demux2/2 -> Mux3/2, SteamflowOutAttemp1/1, Mux5/2
  Boiler Pressure/1 -> Mux5/1, Mux3/1, Mux2/1
  Steamflowboiler/1 -> Mux2/2
  Ts_Out2/1 -> Mux2/3
  attemp_flow3/1 -> Temperature Control2/2(AttempSS)  "Attemp flow SS"
  Demux2/1 -> Temperature Control2/1(Ts_OutAttemp1), Ts_OutAttemp1/1, Mux3/4
  Temperature Control2/1(Attemp_flow_controlled) -> Mux2/4
  Demux4/1 -> Mux3/5, TFG_Out3/1, Scope4/1  "TFG_out3"
  TFG_out5/1 -> Mux1/2
  Superheater3_FG/1 -> Demux4/1
  Demux1/1 -> Mux4/2, Mux5/5, TFG_Out4/1, Scope5/1  "TFG_out4"
  Superheater1/1 -> Demux1/1
  Demux3/1 -> Temperature Control2/3(Ts_Out4), Mux1/4, Ts_Out4/1
  Demux1/2 -> Scope6/1  "Q (kW)"
  Superheater3_Steam/1 -> Mux4/4, Mux5/4, Ts_Out3/1
  U-Value/1 -> Mux3/3, Mux4/3, Mux5/3, Mux1/3
  Demux4/2 -> Scope7/1  "Q (kW)"
  FG_flow/1 -> Mux4/1, Mux1/1
  Mux4/1 -> Superheater3_FG/1
  Mux1/1 -> Superheater1/1

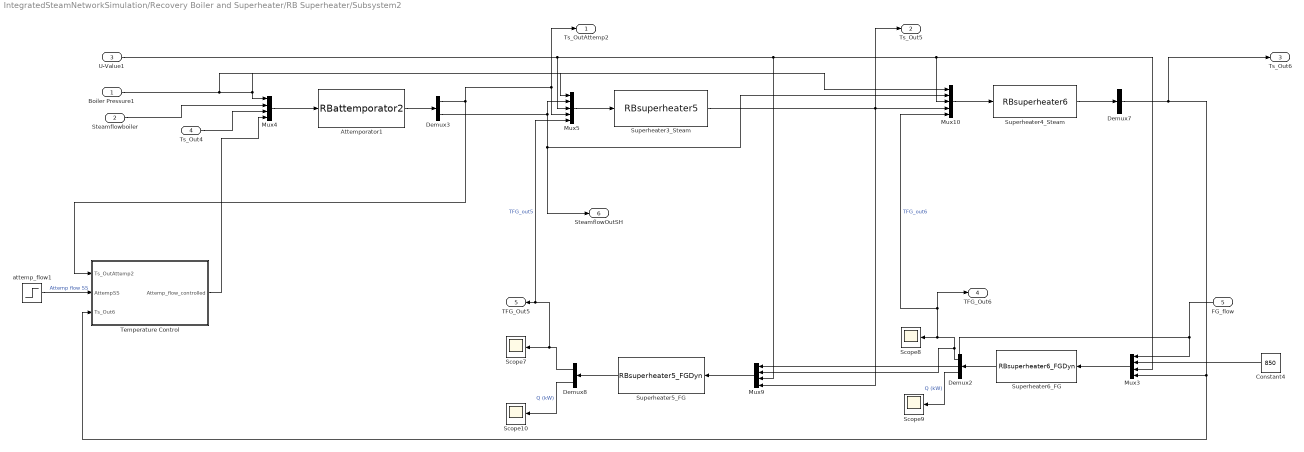
== system IntegratedSteamNetworkSimulation/Recovery Boiler and Superheater/RB Superheater/Subsystem2 ==
  Boiler Pressure1 : Inport
  Steamflowboiler : Inport  Port=2
  U-Value1 : Inport  Port=3
  Ts_Out4 : Inport  Port=4
  FG_flow : Inport  Port=5
  Attemporator1 : S-Function  FunctionName=RBattemporator2  Parameters=Param4,Attemp2_RB  SFunctionDeploymentMode=off  EnableBusSupport=off
  Constant4 : Constant  Value=850
  Demux2 : Demux  Outputs=2
  Demux3 : Demux  Outputs=2
  Demux7 : Demux  Outputs=1
  Demux8 : Demux  Outputs=2
  Mux10 : Mux  Inputs=5
  Mux3 : Mux
  Mux4 : Mux
  Mux5 : Mux  Inputs=5
  Mux9 : Mux
  Scope{7..10} (4 alike) : Scope
  Superheater3_Steam : S-Function  FunctionName=RBsuperheater5  Parameters=Param4,Ts_out5_init_RB  SFunctionDeploymentMode=off  EnableBusSupport=off
  Superheater4_Steam : S-Function  FunctionName=RBsuperheater6  Parameters=Param4,Ts_out6_init_RB  SFunctionDeploymentMode=off  EnableBusSupport=off
  Superheater5_FG : S-Function  FunctionName=RBsuperheater5_FGDyn  Parameters=Param6,TFG_out5_initRB  SFunctionDeploymentMode=off  EnableBusSupport=off
  Superheater6_FG : S-Function  FunctionName=RBsuperheater6_FGDyn  Parameters=Param6,TFG_out6_initRB  SFunctionDeploymentMode=off  EnableBusSupport=off
  Temperature Control : Subsystem
  attemp_flow1 : Step  Time=100  Before=Attempflow_init  After=Attempflow_init  SampleTime=0
  Ts_OutAttemp2 : Outport
  Ts_Out5 : Outport  Port=2
  Ts_Out6 : Outport  Port=3
  TFG_Out6 : Outport  Port=4
  TFG_Out5 : Outport  Port=5
  SteamflowOutSH : Outport  Port=6
  wires:
  Demux8/1 -> Mux5/5, TFG_Out5/1, Scope7/1  "TFG_out5"
  Demux3/1 -> Temperature Control/1(Ts_OutAttemp2), Ts_OutAttemp2/1, Mux5/4
  Superheater5_FG/1 -> Demux8/1
  Superheater6_FG/1 -> Demux2/1
  Mux4/1 -> Attemporator1/1
  Constant4/1 -> Mux3/2
  Temperature Control/1(Attemp_flow_controlled) -> Mux4/4
  Demux7/1 -> Temperature Control/3(Ts_Out6), Mux3/4, Ts_Out6/1
  Demux3/2 -> Mux5/2, SteamflowOutSH/1, Mux10/2
  Demux8/2 -> Scope10/1  "Q (kW)"
  Mux9/1 -> Superheater5_FG/1
  FG_flow/1 -> Mux9/1, Mux3/1
  Demux2/2 -> Scope9/1  "Q (kW)"
  U-Value1/1 -> Mux5/3, Mux9/3, Mux10/3, Mux3/3
  Mux3/1 -> Superheater6_FG/1
  Superheater3_Steam/1 -> Mux9/4, Mux10/4, Ts_Out5/1
  Demux2/1 -> Mux9/2, Mux10/5, TFG_Out6/1, Scope8/1  "TFG_out6"
  Superheater4_Steam/1 -> Demux7/1
  attemp_flow1/1 -> Temperature Control/2(AttempSS)  "Attemp flow SS"
  Mux5/1 -> Superheater3_Steam/1
  Ts_Out4/1 -> Mux4/3
  Boiler Pressure1/1 -> Mux10/1, Mux5/1, Mux4/1
  Steamflowboiler/1 -> Mux4/2
  Mux10/1 -> Superheater4_Steam/1
  Attemporator1/1 -> Demux3/1

== system IntegratedSteamNetworkSimulation/Recovery Boiler and Superheater/Recovery Boiler/3 Element Level Control System ==
  In1 : Inport
  In2 : Inport  Port=2
  Add1 : Sum  Inputs=+-
  Bias : Constant  Value=50
  FB Level Control : Subsystem
  FF Gain : Gain  SaturateOnIntegerOverflow=on  OutDataTypeStr=Inherit: Same as input  ParamDataTypeStr=Inherit: Same as input
  Level Setpoint : Constant  Value=2
  Nominal : Step  Time=10  Before=qfsteadystate  After=qfsteadystate  SampleTime=0
  Real Output from CO : Gain  Gain=10  SaturateOnIntegerOverflow=on  OutDataTypeStr=Inherit: Same as input  ParamDataTypeStr=Inherit: Same as input
  Sum3 : Sum  Inputs=|++-  InputSameDT=on  SaturateOnIntegerOverflow=on  OutDataTypeStr=Inherit: Same as first input
  conversion : Gain  Gain=1000/2.2/3600  SaturateOnIntegerOverflow=on  OutDataTypeStr=Inherit: Same as input  ParamDataTypeStr=Inherit: Same as input
  conversion1 : Gain  Gain=1/(1000/2.2/3600)  SaturateOnIntegerOverflow=on  OutDataTypeStr=Inherit: Same as input  ParamDataTypeStr=Inherit: Same as input
  scaling : Gain  Gain=1/10  SaturateOnIntegerOverflow=on  OutDataTypeStr=Inherit: Same as input  ParamDataTypeStr=Inherit: Same as input
  Delta qf : Outport
  wires:
  In2/1 -> conversion1/1
  Level Setpoint/1 -> FB Level Control/1(In1)
  In1/1 -> FB Level Control/2(In2)
  FB Level Control/1(Out1) -> Sum3/1
  Sum3/1 -> Real Output from CO/1
  Real Output from CO/1 -> conversion/1
  conversion1/1 -> scaling/1
  Bias/1 -> Sum3/3
  scaling/1 -> FF Gain/1
  conversion/1 -> Add1/1
  Nominal/1 -> Add1/2
  FF Gain/1 -> Sum3/2
  Add1/1 -> Delta qf/1

== system IntegratedSteamNetworkSimulation/Recovery Boiler and Superheater/Recovery Boiler/Recovery Boiler ==
  Delta qf : Inport
  Delta Q : Inport  Port=2
  Bias : Bias  Bias=-0.64  SaturateOnIntegerOverflow=off
  FireSide Dyn. : TransferFcn  Denominator=[5 1]
  Recovery Boiler : Subsystem
  Transport Delay : TransportDelay  DelayTime=10
  conversion : Gain  Gain=100/2.54  SaturateOnIntegerOverflow=on  OutDataTypeStr=Inherit: Same as input  ParamDataTypeStr=Inherit: Same as input
  conversion1 : Gain  Gain=1/6.9e3  SaturateOnIntegerOverflow=on  OutDataTypeStr=Inherit: Same as input  ParamDataTypeStr=Inherit: Same as input
  conversion2 : Gain  Gain=2.2*3600/1000  SaturateOnIntegerOverflow=on  OutDataTypeStr=Inherit: Same as input  ParamDataTypeStr=Inherit: Same as input
  l : Outport
  qsf : Outport  Port=2
  RB p : Outport  Port=3
  qf : Outport  Port=4
  wires:
  Delta qf/1 -> Recovery Boiler/1(In2)
  conversion/1 -> l/1
  FireSide Dyn./1 -> Recovery Boiler/2(In3)
  Bias/1 -> conversion/1
  conversion1/1 -> RB p/1
  Transport Delay/1 -> FireSide Dyn./1
  Delta Q/1 -> Transport Delay/1
  conversion2/1 -> qf/1
  Recovery Boiler/1(Out2) -> Bias/1
  Recovery Boiler/2(Out1) -> qsf/1
  Recovery Boiler/3(Out3) -> conversion1/1
  Recovery Boiler/4(Out4) -> conversion2/1

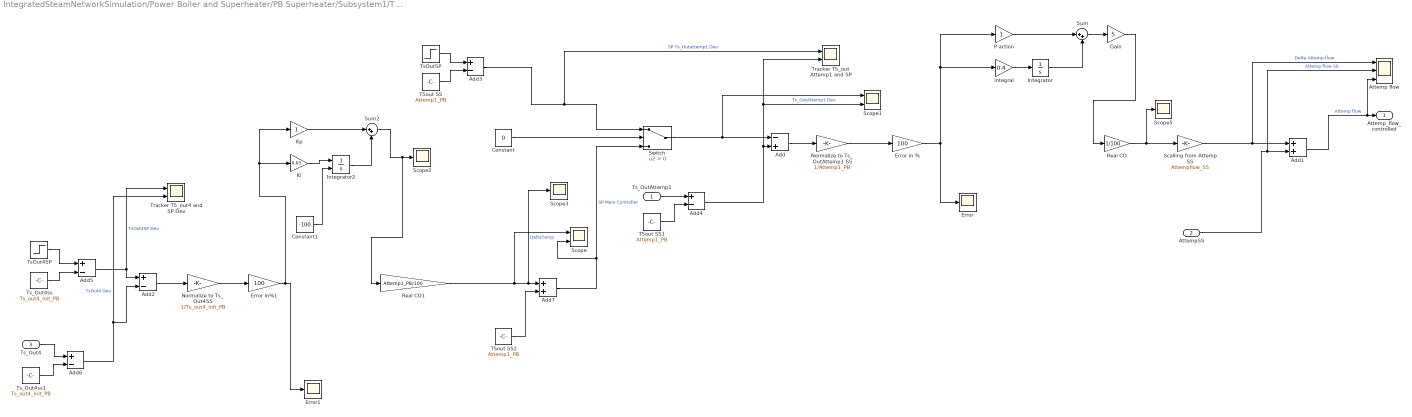
== system IntegratedSteamNetworkSimulation/Power Boiler and Superheater/PB Superheater/Subsystem1/Temperature Control ==
  Ts_OutAttemp1 : Inport
  AttempSS : Inport  Port=2
  Ts_Out4 : Inport  Port=3
  Add : Sum  Inputs=-+
  Add1 : Sum
  Add{2..6} (5 alike) : Sum  Inputs=+-
  Add7 : Sum
  Attemp flow : Scope  NumInputPorts=3
  Constant : Constant  Value=0
  Constant1 : Constant  Value=-100
  Error : Scope
  Error in % : Gain  Gain=100
  Error in%1 : Gain  Gain=100
  Error1 : Scope
  Gain : Gain  Gain=5
  Integrator : Integrator
  Integrator2 : Integrator  InitialConditionSource=external  InitialCondition=-100.1
  Ki : Gain  Gain=0.03
  Kp : Gain
  Normalize to Ts_Out4SS : Gain  Gain=1/Ts_out4_init_PB
  Normalize to Ts_OutAttemp1 SS : Gain  Gain=1/Attemp1_PB
  P action : Gain
  Real CO : Gain  Gain=1/100
  Real CO1 : Gain  Gain=Attemp1_PB/100
  Scalling from Attemp SS : Gain  Gain=Attempflow_SS
  Scope : Scope  NumInputPorts=2
  Scope1 : Scope  NumInputPorts=2
  Scope2 : Scope
  Scope3 : Scope
  Scope5 : Scope
  Sum : Sum  Inputs=|++
  Sum2 : Sum  Inputs=|++
  Switch : Switch  Criteria=u2 > Threshold  SaturateOnIntegerOverflow=off  InputSameDT=off
  TSout SS : Constant  Value=Attemp1_PB
  TSout SS1 : Constant  Value=Attemp1_PB
  TSout SS2 : Constant  Value=Attemp1_PB
  Tracker TS_out Attemp1 and SP : Scope  NumInputPorts=2
  Tracker TS_out4 and SP Dev : Scope  NumInputPorts=2
  TsOut4SP : Step  Time=5000  Before=Ts_out4_init_PB  After=416  SampleTime=0
  TsOutSP : Step  Time=50  Before=Attemp1_PB  After=340  SampleTime=0
  Ts_Out4ss : Constant  Value=Ts_out4_init_PB
  Ts_Out4ss1 : Constant  Value=Ts_out4_init_PB
  integral : Gain  Gain=0.4
  Attemp_flow_controlled : Outport
  wires:
  Add1/1 -> Attemp flow/3, Attemp_flow_controlled/1  "Attemp flow"
  AttempSS/1 -> Attemp flow/2, Add1/2  "Attemp flow SS"
  TsOutSP/1 -> Add3/1
  TSout SS/1 -> Add3/2
  Ts_OutAttemp1/1 -> Add4/1
  TSout SS1/1 -> Add4/2
  Switch/1 -> Scope1/1, Add/1
  Add4/1 -> Tracker TS_out Attemp1 and SP/2, Scope1/2, Add/2  "Ts_OutAttemp1 Dev"
  Add3/1 -> Tracker TS_out Attemp1 and SP/1, Switch/1  "SP Ts_Outattemp1 Dev"
  Constant/1 -> Switch/2
  TsOut4SP/1 -> Add5/1
  Ts_Out4ss/1 -> Add5/2
  Add5/1 -> Tracker TS_out4 and SP Dev/1, Add2/1  "TsOut4SP Dev"
  Ts_Out4/1 -> Add6/1
  Ts_Out4ss1/1 -> Add6/2
  Add6/1 -> Add2/2, Tracker TS_out4 and SP Dev/2  "TsOut4 Dev"
  Real CO1/1 -> Scope/1, Add7/1, Scope3/1  "DeltaTemp"
  TSout SS2/1 -> Add7/2
  Add7/1 -> Scope/2, Switch/3  "SP Main Controller"
  Add/1 -> Normalize to Ts_OutAttemp1 SS/1
  Normalize to Ts_OutAttemp1 SS/1 -> Error in %/1
  Scalling from Attemp SS/1 -> Add1/1, Attemp flow/1  "Delta Attemp flow"
  Add2/1 -> Normalize to Ts_Out4SS/1
  Normalize to Ts_Out4SS/1 -> Error in%1/1
  Real CO/1 -> Scope5/1, Scalling from Attemp SS/1
  Ki/1 -> Integrator2/1
  Integrator2/1 -> Sum2/2
  Constant1/1 -> Integrator2/2
  Sum2/1 -> Real CO1/1, Scope2/1
  Kp/1 -> Sum2/1
  Error in%1/1 -> Error1/1, Kp/1, Ki/1
  Integrator/1 -> Sum/2
  P action/1 -> Sum/1
  Error in %/1 -> P action/1, integral/1, Error/1
  integral/1 -> Integrator/1
  Sum/1 -> Gain/1
  Gain/1 -> Real CO/1

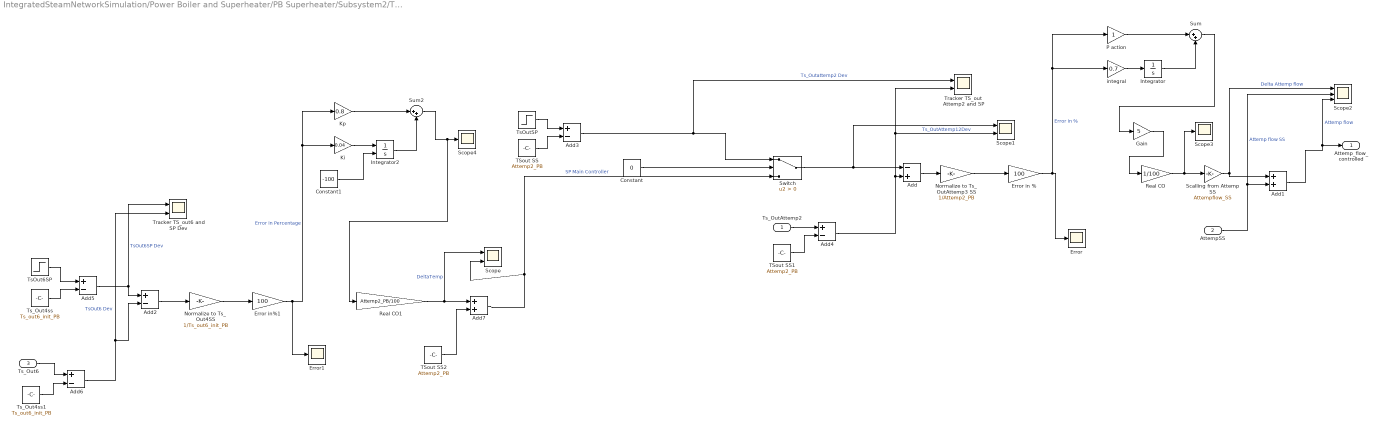
== system IntegratedSteamNetworkSimulation/Power Boiler and Superheater/PB Superheater/Subsystem2/Temperature Control1 ==
  Ts_OutAttemp2 : Inport
  AttempSS : Inport  Port=2
  Ts_Out6 : Inport  Port=3
  Add : Sum  Inputs=-+
  Add1 : Sum
  Add{2..6} (5 alike) : Sum  Inputs=+-
  Add7 : Sum
  Constant : Constant  Value=0
  Constant1 : Constant  Value=-100
  Error : Scope
  Error in % : Gain  Gain=100
  Error in%1 : Gain  Gain=100
  Error1 : Scope
  Gain : Gain  Gain=5
  Integrator : Integrator
  Integrator2 : Integrator  InitialConditionSource=external  InitialCondition=-100.1
  Ki : Gain  Gain=0.04
  Kp : Gain  Gain=0.8
  Normalize to Ts_Out4SS : Gain  Gain=1/Ts_out6_init_PB
  Normalize to Ts_OutAttemp3 SS : Gain  Gain=1/Attemp2_PB
  P action : Gain
  Real CO : Gain  Gain=1/100
  Real CO1 : Gain  Gain=Attemp2_PB/100
  Scalling from Attemp SS : Gain  Gain=Attempflow_SS
  Scope : Scope  NumInputPorts=2
  Scope1 : Scope  NumInputPorts=2
  Scope2 : Scope  NumInputPorts=3
  Scope3 : Scope
  Scope4 : Scope
  Sum : Sum  Inputs=|++
  Sum2 : Sum  Inputs=|++
  Switch : Switch  Criteria=u2 > Threshold  SaturateOnIntegerOverflow=off  InputSameDT=off
  TSout SS : Constant  Value=Attemp2_PB
  TSout SS1 : Constant  Value=Attemp2_PB
  TSout SS2 : Constant  Value=Attemp2_PB
  Tracker TS_out Attemp2 and SP : Scope  NumInputPorts=2
  Tracker TS_out6 and SP Dev : Scope  NumInputPorts=2
  TsOut6SP : Step  Time=50000  Before=Ts_out6_init_PB  After=540  SampleTime=0
  TsOutSP : Step  Time=50  Before=Attemp2_PB  After=442  SampleTime=0
  Ts_Out4ss : Constant  Value=Ts_out6_init_PB
  Ts_Out4ss1 : Constant  Value=Ts_out6_init_PB
  integral : Gain  Gain=0.7
  Attemp_flow_controlled : Outport
  wires:
  Normalize to Ts_Out4SS/1 -> Error in%1/1
  TsOutSP/1 -> Add3/1
  AttempSS/1 -> Scope2/2, Add1/2  "Attemp flow SS"
  Scalling from Attemp SS/1 -> Scope2/1, Add1/1  "Delta Attemp flow"
  Normalize to Ts_OutAttemp3 SS/1 -> Error in %/1
  Add7/1 -> Scope/2, Switch/3  "SP Main Controller"
  Add4/1 -> Tracker TS_out Attemp2 and SP/2, Scope1/2, Add/2  "Ts_OutAttemp12Dev"
  Add/1 -> Normalize to Ts_OutAttemp3 SS/1
  Add2/1 -> Normalize to Ts_Out4SS/1
  Error in %/1 -> Error/1, P action/1, integral/1  "Error in %"
  Switch/1 -> Scope1/1, Add/1
  TSout SS1/1 -> Add4/2
  Real CO1/1 -> Add7/1, Scope/1  "DeltaTemp"
  Add5/1 -> Tracker TS_out6 and SP Dev/1, Add2/1  "TsOut6SP Dev"
  Ts_Out4ss/1 -> Add5/2
  Ts_OutAttemp2/1 -> Add4/1
  Ts_Out4ss1/1 -> Add6/2
  Add3/1 -> Tracker TS_out Attemp2 and SP/1, Switch/1  "Ts_Outattemp2 Dev"
  TsOut6SP/1 -> Add5/1
  Constant/1 -> Switch/2
  Add1/1 -> Scope2/3, Attemp_flow_controlled/1  "Attemp flow"
  Error in%1/1 -> Kp/1, Ki/1, Error1/1  "Error in Percentage"
  TSout SS2/1 -> Add7/2
  Add6/1 -> Add2/2, Tracker TS_out6 and SP Dev/2  "TsOut6 Dev"
  Ts_Out6/1 -> Add6/1
  TSout SS/1 -> Add3/2
  Real CO/1 -> Scope3/1, Scalling from Attemp SS/1
  Constant1/1 -> Integrator2/2
  Sum2/1 -> Real CO1/1, Scope4/1
  Ki/1 -> Integrator2/1
  Kp/1 -> Sum2/1
  Integrator2/1 -> Sum2/2
  integral/1 -> Integrator/1
  Integrator/1 -> Sum/2
  P action/1 -> Sum/1
  Sum/1 -> Gain/1
  Gain/1 -> Real CO/1

== system IntegratedSteamNetworkSimulation/Power Boiler and Superheater/Power Boiler/3 Element Level Control System/FB Level Control ==
  In1 : Inport
  In2 : Inport  Port=2
  1/Ti1 : Gain  Gain=1/3/60  SaturateOnIntegerOverflow=on  OutDataTypeStr=Inherit: Same as input  ParamDataTypeStr=Inherit: Same as input
  Bias : Constant  Value=50
  Integrator1 : Integrator
  Kc1 : Gain  Gain=1.38  SaturateOnIntegerOverflow=on  OutDataTypeStr=Inherit: Same as input  ParamDataTypeStr=Inherit: Same as input
  P action1 : Gain  SaturateOnIntegerOverflow=on  OutDataTypeStr=Inherit: Same as input  ParamDataTypeStr=Inherit: Same as input
  Sum1 : Sum  Inputs=|++  InputSameDT=on  SaturateOnIntegerOverflow=on  OutDataTypeStr=Inherit: Same as first input
  Sum2 : Sum  Inputs=|++  InputSameDT=on  SaturateOnIntegerOverflow=on  OutDataTypeStr=Inherit: Same as first input
  Sum4 : Sum  Inputs=|+-  InputSameDT=on  SaturateOnIntegerOverflow=on  OutDataTypeStr=Inherit: Same as first input
  error as % of Range : Gain  Gain=100/25  SaturateOnIntegerOverflow=on  OutDataTypeStr=Inherit: Same as input  ParamDataTypeStr=Inherit: Same as input
  Out1 : Outport
  wires:
  1/Ti1/1 -> Integrator1/1
  P action1/1 -> Sum1/1
  Integrator1/1 -> Sum1/2
  error as % of Range/1 -> 1/Ti1/1, P action1/1
  Sum4/1 -> error as % of Range/1
  In1/1 -> Sum4/1
  In2/1 -> Sum4/2
  Sum2/1 -> Out1/1
  Bias/1 -> Sum2/2
  Kc1/1 -> Sum2/1
  Sum1/1 -> Kc1/1

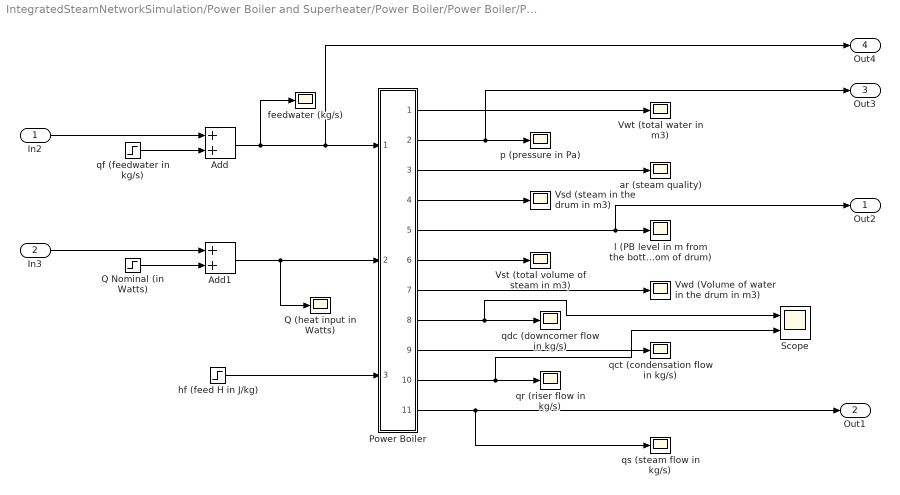
== system IntegratedSteamNetworkSimulation/Power Boiler and Superheater/Power Boiler/Power Boiler/Power Boiler ==
  In2 : Inport
  In3 : Inport  Port=2
  Add : Sum
  Add1 : Sum
  Power Boiler : Subsystem
      mask Display: disp('')
  Q (heat input in Watts) : Scope
  Q Nominal (in Watts) : Step  Time=10  Before=5.9194e7  After=5.9194e7  SampleTime=0
  Scope : Scope  NumInputPorts=2
  Vsd (steam in the drum in m3) : Scope
  Vst (total volume of steam in m3) : Scope
  Vwd (Volume of water in the drum in m3) : Scope
  Vwt (total water in m3) : Scope
  ar (steam quality) : Scope
  feedwater (kg/s) : Scope
  hf (feed H in J/kg) : Step  Time=50  Before=hf  After=hf  SampleTime=0
  l (PB level in m from the bottom of drum) : Scope
  "p (pressure in Pa) " : Scope
  qct (condensation flow in kg/s) : Scope
  qdc (downcomer flow in kg/s) : Scope
  qf (feedwater in kg/s) : Step  Time=20  Before=31.5679  After=31.5679  SampleTime=0
  qr (riser flow in kg/s) : Scope
  qs (steam flow in kg/s) : Scope
  Out2 : Outport
  Out1 : Outport  Port=2
  Out3 : Outport  Port=3
  Out4 : Outport  Port=4
  wires:
  hf (feed H in J/kg)/1 -> Power Boiler/3(In4)
  qf (feedwater in kg/s)/1 -> Add/2
  Q Nominal (in Watts)/1 -> Add1/2
  Add1/1 -> Power Boiler/2(In3), Q (heat input in Watts)/1
  Add/1 -> Power Boiler/1(In1), Out4/1, feedwater (kg/s)/1
  Power Boiler/6(Out6) -> Vst (total volume of steam in m3)/1
  Power Boiler/10(Out10) -> Scope/2, qr (riser flow in kg/s)/1
  Power Boiler/9(Out9) -> qct (condensation flow in kg/s)/1
  Power Boiler/8(Out8) -> Scope/1, qdc (downcomer flow in kg/s)/1
  Power Boiler/7(Out7) -> Vwd (Volume of water in the drum in m3)/1
  Power Boiler/5(Out5) -> Out2/1, l (PB level in m from the bottom of drum)/1
  Power Boiler/4(Out4) -> Vsd (steam in the drum in m3)/1
  Power Boiler/3(Out3) -> ar (steam quality)/1
  Power Boiler/2(Out2) -> "p (pressure in Pa) "/1, Out3/1
  Power Boiler/1(Out1) -> Vwt (total water in m3)/1
  In3/1 -> Add1/1
  Power Boiler/11(Out11) -> Out1/1, qs (steam flow in kg/s)/1
  In2/1 -> Add/1
